simulink model "dsc_pid_2026a"  (R2026a)
settings: Solver=FixedStepAuto  StopTime=5  FixedStep=0.001  EnableMultiTasking=on
libraries: stm32f4xxblockslib x3, dspstat3 x2, stm32blockslib x1
settings Model: STM32="{\"EncoderBlock\":{\"ID\":\"1\"},\"PWMOutput\":{\"ID\":\"2\"},\"DigitalPortWrite\":[{\"ID\":\"5\"},{\"ID\":\"6\"}]}"  Creator=drbha  LastModifiedBy=drbha
settings OptimizationCC: MaxStackSize=512
settings HardwareCC: ProdLargestAtomicInteger=Long  ProdLargestAtomicFloat=Double  ProdHWDeviceType=ARM Compatible->ARM Cortex-M
settings SFSimCC: SimGPUStackLimitPerThread=51200
settings RTWCC: GPUStackLimitPerThread=51200  SystemTargetFile=ert.tlc  HardwareBoard=STM32F4xx Based  TLCOptions=-aInlineSetEventsForThisBaseRateFcn=TLC_FALSE -aSuppressMultiTaskScheduler=TLC_FALSE -aRateBasedStepFcn=1  Toolchain=GNU Tools for STM32  BuildConfiguration=Faster Runs  Description=Embedded Coder
settings ERTTargetCC: ExtModeTransport=3.0  ExtModeStaticAllocSize=2048.0  CodeReplacementLibrary=ARM Cortex-M  CombineSignalStateStructs=on

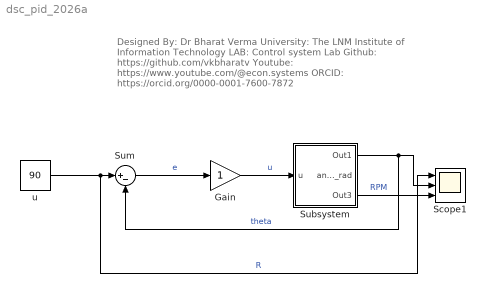
== system dsc_pid_2026a ==
  note: Designed By: Dr Bharat Verma
      | University: The LNM Institute of Information Technology
      | LAB: Control system Lab
      | Github: https://github.com/vkbharatv
      | Youtube: https://www.youtube.com/@econ.systems
      | ORCID: https://orcid.org/0000-0001-7600-7872
  Gain : Gain
  Scope1 : Scope  NumInputPorts=3
      settings: ActiveDisplayYMinimum=-40.151692481390207  ActiveDisplayYMaximum=143.29912140932385
  Subsystem : Subsystem
  Sum : Sum  Inputs=|+-
  u : Constant  Value=90
  wires:
  Sum/1 -> Gain/1  "e"
  Subsystem/1(Out1) -> Sum/2, Scope1/2  "theta"
  u/1 -> Scope1/1, Sum/1  "R"
  Gain/1 -> Subsystem/1(u)  "u"
  Subsystem/3(Out3) -> Scope1/3  "RPM"

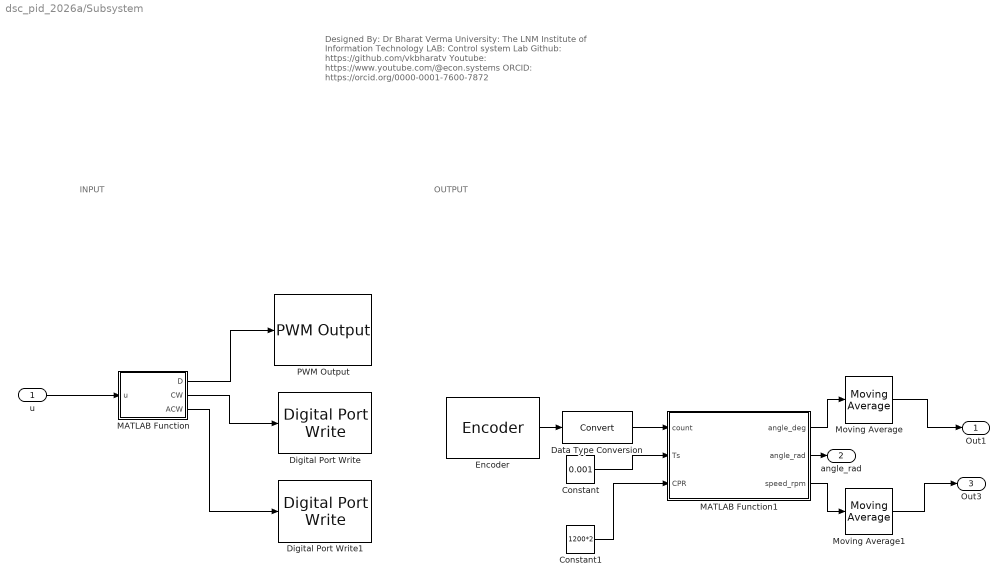
== system dsc_pid_2026a/Subsystem ==
  note: Designed By: Dr Bharat Verma
      | University: The LNM Institute of Information Technology
      | LAB: Control system Lab
      | Github: https://github.com/vkbharatv
      | Youtube: https://www.youtube.com/@econ.systems
      | ORCID: https://orcid.org/0000-0001-7600-7872
  note: OUTPUT
  note: INPUT
  u : Inport
  Constant : Constant  Value=0.001
  Constant1 : Constant  Value=1200*2
  Data Type Conversion : DataTypeConversion  SaturateOnIntegerOverflow=off  RndMeth=Floor
  Digital Port Write : stm32f4xxblockslib/Digital Port Write  PortName=GPIOA  PinNumber=[9]  ReadOperation=off  IOAsArray=on  EnableSimPort=off  hoistedMaskSrc=ECSoC/ECSimCodegen/Digital Port Write
  Digital Port Write1 : stm32f4xxblockslib/Digital Port Write  PortName=GPIOC  PinNumber=[7]  ReadOperation=off  IOAsArray=on  EnableSimPort=off  hoistedMaskSrc=ECSoC/ECSimCodegen/Digital Port Write
  Encoder : stm32blockslib/Encoder  TimerModule=TIM2  EnableResetInput=off  OutputDirection=off  SampleTime=-1
      settings: LibrarySourceBlock=stm32f4xxblockslib/Encoder
  MATLAB Function : MATLAB Function  TreatAsAtomicUnit=on
  MATLAB Function1 : MATLAB Function  TreatAsAtomicUnit=on
  Moving Average : dspstat3/Moving Average  Method=Exponential weighting  ForgettingFactorPort=off  SpecifyWindowLength=on  WindowLengthSource=Property  MaxWindowLength=20  WindowLength=4  OverlapLength=3  AllowArbitraryInputLength=off  ForgettingFactor=0.95  SimulateUsing=Interpreted execution
  Moving Average1 : dspstat3/Moving Average  Method=Exponential weighting  ForgettingFactorPort=off  SpecifyWindowLength=on  WindowLengthSource=Property  MaxWindowLength=20  WindowLength=4  OverlapLength=3  AllowArbitraryInputLength=off  ForgettingFactor=0.99  SimulateUsing=Interpreted execution
  PWM Output : stm32f4xxblockslib/PWM Output  ProcessorFamily=STM32F4  TimerModule=TIM1  DutycycleUnits=Percentage  EnableChannel1=on  EnableCaptureCompare1Input=off  EnableCaptureCompare1ComplementaryInput=off  EnableOutputCompare1ModeInput=off  EnableChannel2=off  EnableCaptureCompare2Input=off  EnableCaptureCompare2ComplementaryInput=off  EnableOutputCompare2ModeInput=off  EnableChannel3=off  EnableCaptureCompare3Input=off  EnableCaptureCompare3ComplementaryInput=off  EnableOutputCompare3ModeInput=off  EnableChannel4=off  EnableCaptureCompare4Input=off  EnableCaptureCompare4ComplementaryInput=off  EnableOutputCompare4ModeInput=off  EnableChannel5=off  EnableCaptureCompare5Input=off  EnableOutputCompare5ModeInput=off  EnableChannel6=off  EnableCaptureCompare6Input=off  EnableOutputCompare6ModeInput=off  EnableCounterInput=off  EnableMainOutputInput=off  EnableFrequencyInput=off  SetRCAfterCE=off  OutputDirection=off  OutputMainOutputEnableStatus=off  SampleTime=0.1  EnableSimPort=off  EnableUpdateEvent=off  EnableCaptureCompare1Event=off  EnableCaptureCompare2Event=off  EnableCaptureCompare3Event=off  EnableCaptureCompare4Event=off  EnableTriggerEvent=off  EnableBreakEvent=off  EnableBreakEvent2=off  hoistedMaskSrc=ECSoC/ECSimCodegen/PWM Output
  Out1 : Outport
  angle_rad : Outport  Port=2
  Out3 : Outport  Port=3
  wires:
  Moving Average1/1 -> Out3/1
  MATLAB Function/1(D) -> PWM Output/1
  MATLAB Function1/3(speed_rpm) -> Moving Average1/1
  MATLAB Function/2(CW) -> Digital Port Write/1
  Encoder/1 -> Data Type Conversion/1
  MATLAB Function/3(ACW) -> Digital Port Write1/1
  Constant/1 -> MATLAB Function1/2(Ts)
  MATLAB Function1/1(angle_deg) -> Moving Average/1
  Data Type Conversion/1 -> MATLAB Function1/1(count)
  Constant1/1 -> MATLAB Function1/3(CPR)
  u/1 -> MATLAB Function/1(u)
  Moving Average/1 -> Out1/1
  MATLAB Function1/2(angle_rad) -> angle_rad/1

== matlab function dsc_pid_2026a/Subsystem/MATLAB Function1 ==
  data: count input; angle_deg output; Ts input; CPR input; angle_rad output; speed_rpm output
function [angle_deg, angle_rad, speed_rpm] = encoder_angle(count, Ts, CPR)

CPR = int64(CPR);

persistent last_count
persistent total_count

if isempty(last_count)
    last_count = int64(count);
    total_count = int64(0);
end

current_count = int64(count);

delta = current_count - last_count;

if delta > int64(2147483648)
    delta = delta - int64(4294967296);
elseif delta < int64(-2147483648)
    delta = delta + int64(4294967296);
end

total_count = total_count + delta;

last_count = current_count;

angle_deg = double(total_count) * 360.0 / double(CPR);

angle_rad = double(total_count) * 2.0 * pi / double(CPR);

if Ts > 0
    speed_rpm = double(delta) * 60.0 / ...
        (double(CPR) * Ts);
else
    speed_rpm = 0.0;
end

== matlab function dsc_pid_2026a/Subsystem/MATLAB Function ==
  data: u input; D output; CW output; ACW output
function [D,CW, ACW] = fcn(u)
if u>0
    CW=1;
    ACW=0;
else
    CW=0;
    ACW=1;
end
D = abs(u);
